simulink model "HopperPlant"  (R2023b)
settings: Solver=VariableStepAuto  StartTime=0.0  StopTime=20  RelTol=1e-3
libraries: slpidlib x1
settings Model: Creator=xavie  LastModifiedBy=xavie

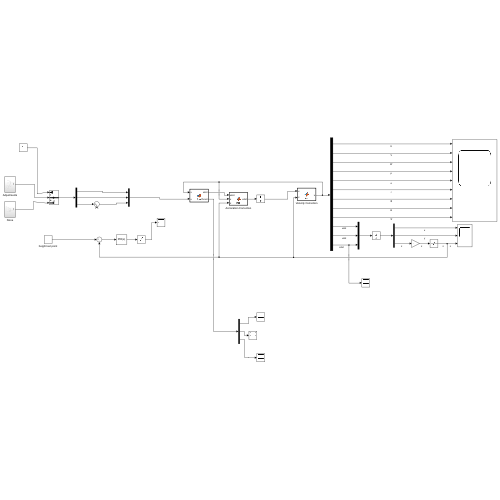
[thumbnail: Simulink's stored preview of the top-level diagram]
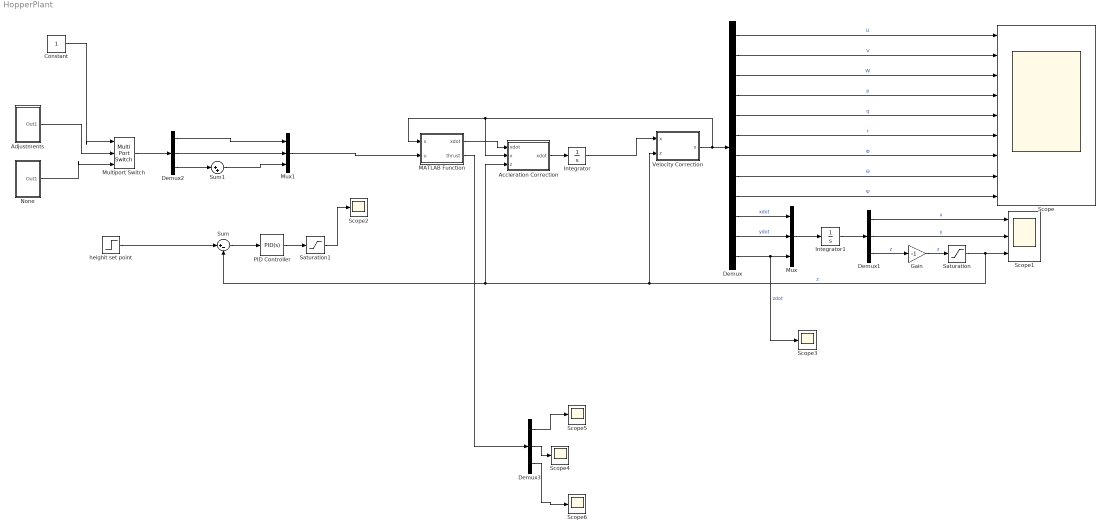
== system HopperPlant ==
  Accleration Correction : MATLAB Function  TreatAsAtomicUnit=on
  Adjustments : Subsystem
  Constant : Constant
  Demux : Demux  Outputs=12
  Demux1 : Demux  Outputs=3
  Demux2 : Demux  Outputs=3
  Demux3 : Demux  Outputs=3
  Gain : Gain  Gain=-1
  Integrator : Integrator  InitialCondition=[0;0;0;0;0;0;0;0;0;0;0;0]
  Integrator1 : Integrator  InitialCondition=[0;0;0]
  MATLAB Function : MATLAB Function  TreatAsAtomicUnit=on
  Multiport Switch : MultiPortSwitch  Inputs=2  SaturateOnIntegerOverflow=off  InputSameDT=off
  Mux : Mux  Inputs=3
  Mux1 : Mux  Inputs=3
  None : Subsystem
  PID Controller : slpidlib/PID Controller  Controller=PID  Form=Parallel  TimeDomain=Continuous-time  UseExternalTs=off  SampleTime=-1  IntegratorMethod=Forward Euler  FilterMethod=Forward Euler  ControllerParametersSource=internal  P=12  I=1.2  UseKiTs=off  D=30  N=100  UseFilter=on  TunerSelectOption=Transfer Function Based (PID Tuner App)  InitialConditionSource=internal  InitialConditionForIntegrator=0  InitialConditionForFilter=0  DifferentiatorICPrevScaledInput=0  ExternalReset=none  TrackingMode=off  Kt=1  LimitOutput=off  SatLimitsSource=internal  UpperSaturationLimit=inf  LowerSaturationLimit=-inf  LinearizeAsGain=on  AntiWindupMode=none  Kb=1  LimitIntegrator=off  UpperIntegratorSaturationLimit=inf  LowerIntegratorSaturationLimit=-inf  POutMin=[]  POutMax=[]  IOutMin=[]  IOutMax=[]  DOutMin=[]  DOutMax=[]  NOutMin=[]  NOutMax=[]  SumOutMin=[]  SumOutMax=[]  SaturationOutMin=[]  SaturationOutMax=[]  PParamMin=[]  PParamMax=[]  IParamMin=[]  IParamMax=[]  DParamMin=[]  DParamMax=[]  NParamMin=[]  NParamMax=[]  KbParamMin=[]  KbParamMax=[]  KtParamMin=[]  KtParamMax=[]  KbOutMin=[]  KbOutMax=[]  KtOutMin=[]  KtOutMax=[]  IntegratorOutMin=[]  IntegratorOutMax=[]  FilterOutMin=[]  FilterOutMax=[]  SumI1OutMin=[]  SumI1OutMax=[]  SumI2OutMin=[]  SumI2OutMax=[]  SumI3OutMin=[]  SumI3OutMax=[]  SumI4OutMin=[]  SumI4OutMax=[]  SumDOutMin=[]  SumDOutMax=[]  DifferentiatorOutMin=[]  DifferentiatorOutMax=[]  FilterDiffOutCoefMin=[]  FilterDiffOutCoefMax=[]  ReciprocalOutMin=[]  ReciprocalOutMax=[]  SumDenOutMin=[]  SumDenOutMax=[]  SumNumOutMin=[]  SumNumOutMax=[]  DivideOutMin=[]  DivideOutMax=[]  UdiffTsProdOutMin=[]  UdiffTsProdOutMax=[]  NTsProdOutMin=[]  NTsProdOutMax=[]  UintegralTsProdOutMin=[]  UintegralTsProdOutMax=[]  UngainTsProdOutMin=[]  UngainTsProdOutMax=[]  ClampingZeroOutDataTypeStr=Inherit: Inherit via back propagation  ClampingZeroOutMin=[]  ClampingZeroOutMax=[]  FilterDenConstantOutDataTypeStr=Inherit: Inherit via back propagation  FilterDenConstantOutMin=[]  FilterDenConstantOutMax=[]  PCopyOutDataTypeStr=Inherit: Inherit via back propagation  PCopyOutMin=[]  PCopyOutMax=[]  NCopyOutDataTypeStr=Inherit: Inherit via back propagation  NCopyOutMin=[]  NCopyOutMax=[]  IntegratorContinuousStateAttributes=''  IntegratorStateMustResolveToSignalObject=off  IntegratorRTWStateStorageClass=Auto  FilterContinuousStateAttributes=''  FilterStateMustResolveToSignalObject=off  FilterRTWStateStorageClass=Auto  ParallelPVariant=InternalParameters  IdealPVariant=Disabled  IVariant=InternalParameters  DVariant=InternalParameters  IntegratorVariant=Continuous  SatVariant=Disabled  AWVariant=Passthrough  PCopyVariant=Disabled  TRVariant=Disabled  FdbkBlocksVariant=Forward  IdealPFdbkVariant=Disabled  SatFdbkVariant=Disabled  DerivativeFilterVariant=ContFilter  NVariant=InternalParameters  NCopyVariant=Disabled  FilterICVariant=InternalICsFilter  IntegratorICVariant=InternalICs  ExternalResetVariant=Disabled  TRSumVariant=Passthrough  SumFdbkVariant=Disabled  SumVariant=Sum_PID  TsampFilterVariant=InternalTs  TsampNgainVariant=Passthrough  TsampIntegralVariant=Disabled_SignalSpec  ExternalSaturationOutDataTypeStr=Inherit: Same as second input
  Saturation : Saturate  UpperLimit=10000000000000000000000000000000000000000000  LowerLimit=0
  Saturation1 : Saturate  UpperLimit=1500  LowerLimit=0
  Scope : Scope  NumInputPorts=9
  Scope1 : Scope  NumInputPorts=3
  Scope{2..6} (5 alike) : Scope
  Sum : Sum  Inputs=|+-
  Sum1 : Sum  Inputs=|++
  Velocity Correction : MATLAB Function  TreatAsAtomicUnit=on
  heighit set point : Step  After=100  SampleTime=0
  wires:
  MATLAB Function/1(xdot) -> Accleration Correction/1("xdot ")
  Integrator/1 -> Velocity Correction/1("x ")
  Demux/1 -> Scope/1  "U"
  Demux/2 -> Scope/2  "V"
  Demux/3 -> Scope/3  "W"
  Demux/4 -> Scope/4  "p"
  Demux/5 -> Scope/5  "q"
  Demux/6 -> Scope/6  "r"
  Demux/7 -> Scope/7  "Φ"
  Demux/8 -> Scope/8  "Θ"
  Demux/9 -> Scope/9  "Ψ"
  Demux/10 -> Mux/1  "xdot"
  Demux/11 -> Mux/2  "ydot"
  Demux/12 -> Scope3/1, Mux/3  "zdot"
  Mux/1 -> Integrator1/1
  Integrator1/1 -> Demux1/1
  Demux1/1 -> Scope1/1  "x"
  Demux1/2 -> Scope1/2  "y"
  Demux1/3 -> Gain/1  "z"
  Gain/1 -> Saturation/1  "z"
  Accleration Correction/1(xdot) -> Integrator/1
  Saturation/1 -> Velocity Correction/2(z), Sum/2, Accleration Correction/3(z), Scope1/3  "z"
  Velocity Correction/1(x) -> Accleration Correction/2(x), MATLAB Function/1(x), Demux/1
  Constant/1 -> Multiport Switch/1
  Adjustments/1(Out1) -> Multiport Switch/2
  None/1(Out1) -> Multiport Switch/3
  heighit set point/1 -> Sum/1
  Sum/1 -> PID Controller/1
  Multiport Switch/1 -> Demux2/1
  Demux2/3 -> Sum1/1
  PID Controller/1 -> Saturation1/1
  Saturation1/1 -> Scope2/1
  Mux1/1 -> MATLAB Function/2(u)
  Sum1/1 -> Mux1/3
  Demux2/2 -> Mux1/2
  Demux2/1 -> Mux1/1
  MATLAB Function/2(thrust) -> Demux3/1
  Demux3/2 -> Scope4/1
  Demux3/1 -> Scope5/1
  Demux3/3 -> Scope6/1

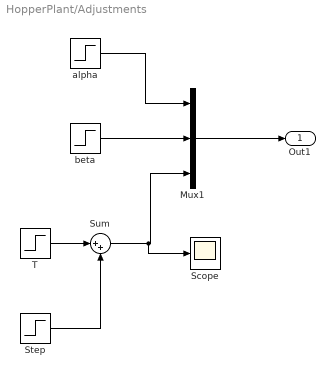
== system HopperPlant/Adjustments ==
  Mux1 : Mux  Inputs=3
  Scope : Scope
  Step : Step  Time=10  After=-1500  SampleTime=0
  Sum : Sum  Inputs=|++
  T : Step  Time=0  After=1500  SampleTime=0
  alpha : Step  Time=0  After=0  SampleTime=0
  beta : Step  Time=0  After=1.553  SampleTime=0
  Out1 : Outport
  wires:
  alpha/1 -> Mux1/1
  Mux1/1 -> Out1/1
  beta/1 -> Mux1/2
  T/1 -> Sum/1
  Step/1 -> Sum/2
  Sum/1 -> Scope/1, Mux1/3

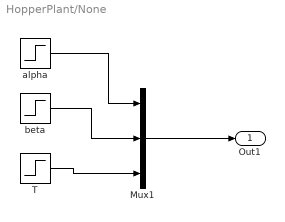
== system HopperPlant/None ==
  Mux1 : Mux  Inputs=3
  T : Step  After=0  SampleTime=0
  alpha : Step  After=0  SampleTime=0
  beta : Step  After=0  SampleTime=0
  Out1 : Outport
  wires:
  beta/1 -> Mux1/2
  T/1 -> Mux1/3
  alpha/1 -> Mux1/1
  Mux1/1 -> Out1/1

== matlab function HopperPlant/Accleration Correction ==
  data: xdot input; x input; xdot output; z input
function xdot = fcn(xdot,x, z)

phi=x(7);
theta=x(8);
psi=x(9);
T_etob=[cos(theta)*cos(psi),cos(theta)*sin(psi),-sin(theta);
    sin(theta)*sin(phi)*cos(phi)-sin(psi)*cos(phi),sin(psi)*sin(theta)*sin(phi)+cos(psi)*cos(phi), sin(phi)*cos(theta);
    sin(theta)*cos(phi)*cos(psi)+sin(psi)*sin(phi), sin(phi)*sin(theta)*cos(phi)-cos(psi)*sin(theta), cos(phi)*cos(theta)];
zddot=xdot(end);

if z <= 0 && zddot > 0
    xdot(end)=0;
    xdot(end-1)=0;
    xdot(end-2)=0;
    xdot(1:3)=T_etob*[xdot(end-2);xdot(end-1);xdot(end)];
    
end

== matlab function HopperPlant/MATLAB Function ==
  data: x input; u input; xdot output; thrust output
function [xdot,thrust]  = fcn(x, u)
%{
Takes in thrust, angles of thrust, x and outputs xdot
Body axis is defined as z being the in the direction of gravity when pitch
is zero

m - mass-kg
I - moment of intertia - kg m^2
cg - centre of gravity - m
thrust position - m
U - body axis x velocity - m/s
V - body axis y velocity - m/s
W - body axis z velocity - m/s
p - body axis roll rate - rad/s
q - body axis pitch rate - rad/s
r - body axis yaw rate - rad/s
phi - earth axis roll - rad
theta - earth axis pitch - rad
psi - earth axis yaw - rad
alpha - thrust rotation angle 
%}


%%Control input
alpha=u(1); 
beta=u(2);
% T1=u(3);
% T2=u(4);
T=u(3);

 % alpha=0; 
 % beta=0;
 % T1=0;
 % T2=0;
 % T=T1+T2;

%%states
U=x(1);
V=x(2);
W=x(3);
p=x(4);
q=x(5);
r=x(6);
phi=x(7);
theta=x(8);
psi=x(9);


%%Constants
T_etob=[cos(theta)*cos(psi), sin(theta)*sin(phi)*cos(psi)-cos(phi)*sin(psi), cos(phi)*sin(theta)*cos(psi)+sin(phi)*sin(psi);
    cos(theta)*sin(psi), sin(phi)*sin(theta)*sin(psi)+cos(phi)*cos(psi), cos(phi)*sin(theta)*cos(psi)-sin(phi)*cos(psi);
    -sin(theta),sin(phi)*cos(theta), cos(phi)*cos(theta)];
gb=9.81;
ge=T_etob*[0;0;gb];
gx=ge(1);
gy=ge(2);
gz=ge(3);

%%Mass and inertia

m=100;
Ixx=units(2.671e10,'g*mm^2','kg*m^2');
Iyy=units(2.671e10,'g*mm^2','kg*m^2');
Izz=units(4.915e09,'g*mm^2','kg*m^2');
Ixz=units(-1.112e06,'g*mm^2','kg*m^2');

% Ixx=units(4.915e09,'g*mm^2','kg*m^2');
% Iyy=units(2.614e10,'g*mm^2','kg*m^2');
% Izz=units(1.614e10,'g*mm^2','kg*m^2');
% Ixz=units(-1.629e08,'g*mm^2','kg*m^2');

cg=[0,0,units(800,'mm','m')];
thrust_pos=[units(0,'mm','m'),0,units(1350,'mm','m')];

%%Forces

 Tx=T*cos(beta)*cos(alpha);
 Ty=T*cos(beta)*sin(alpha);
 Tz=-T*sin(beta);

 Fx=Tx+m*gx;
 Fy=Ty+m*gy;
 Fz=Tz+m*gz;



%%Rotational moments
lx=thrust_pos(1)-cg(1);
ly=thrust_pos(2)-cg(2);
lz=thrust_pos(3)-cg(3);

L=ly*Tz-lz*Ty;
M=lx*Tz+lz*Tx;
N=-lx*Ty-ly*Tx;


%%Compute xdot
Udot=Fx/m-(W*q-V*r);
Vdot=Fy/m-(U*r-p*W);
Wdot=Fz/m-(V*p-U*q);

% A=L+Ixz*q*p-(Izz-Iyy)*q*r;
% B=M-Ixz*(p^2-r^2)-(Ixx-Izz)*p*r;
% C=N-Ixz*q*r-(Iyy-Ixx)*p*q;
% 
% 
% pr_dot=[Ixx, -Ixz; -Ixz, Izz]\[A;C];
% pdot=pr_dot(1);
% qdot=B/Iyy;
% rdot=pr_dot(2);

pdot=(L-q*r*(Izz-Iyy))/Ixx;
qdot=(M-r*p*(Ixx-Izz))/Iyy;
rdot=(N-p*q*(Iyy-Ixx))/Izz;

% Compute Euler angles
AngleCon_btoe=[1 sin(phi)*tan(theta), cos(phi)*tan(theta);
    0, cos(phi), -sin(phi); ...
    0, sin(phi)*sec(theta), cos(phi)*sec(theta)];


EulerAngledot=AngleCon_btoe*[p;q;r];
T_btoe=transpose(T_etob);
Earthacceleration=T_btoe*[Udot;Vdot;Wdot];


xdot=[Udot;Vdot;Wdot;pdot;qdot; rdot;EulerAngledot;Earthacceleration];
thrust=[Fx, Fy, Fz]

== matlab function HopperPlant/Velocity Correction ==
  data: x input; x output; z input
function x = fcn(x, z)

phi=x(7);
theta=x(8);
psi=x(9);
T_etob=[cos(theta)*cos(psi),cos(theta)*sin(psi),-sin(theta);
    sin(theta)*sin(phi)*cos(phi)-sin(psi)*cos(phi),sin(psi)*sin(theta)*sin(phi)+cos(psi)*cos(phi), sin(phi)*cos(theta);
    sin(theta)*cos(phi)*cos(psi)+sin(psi)*sin(phi), sin(phi)*sin(theta)*cos(phi)-cos(psi)*sin(theta), cos(phi)*cos(theta)];
zdot=x(end);

if z <= 0 && zdot > 0
    x(end)=0;
    x(end-1)=0;
    x(end-2)=0;

    x(1:3)=T_etob*[x(end-2);x(end-1);x(end)];
   
end
